simulink library "LocalLib"  (R2015b)
settings: Solver=VariableStepAuto  StartTime=0.0  StopTime=10.0  RelTol=1e-3
values from neighbouring files (symbols this model uses):
  Im = 5e-6    (= 5e-06)    [Params.m]
  Kfr = 5.0e-6    (= 5e-06)    [Params.m]
  KfrOffset = 1.0e-6    (= 1e-06)    [Params.m]
  Ki = (Tq_stall/I_stall)    (= 0.0037456445993)    [MotorModel_Mabuchi_RS_540.m]    (also in Params.m = 0.0041)
  Kv = (Vdc_nom - (I_nl*R_winding))/Om_nl    (= 0.00375385553259)    [MotorModel_Mabuchi_RS_540.m]    (also in Params.m = 0.0039)
  Lm = 1e-5    (= 1e-05)    [Params.m]
  Rm = 0.1672    [Params.m]
libraries: simulink x1
settings Model: Creator=jje  LastModifiedBy=jje

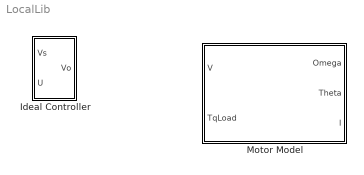
== system LocalLib ==
  Ideal Controller : Subsystem
  Motor Model : Subsystem

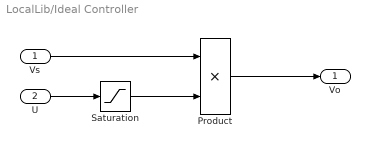
== system LocalLib/Ideal Controller ==
  Vs : Inport
  U : Inport  Port=2
  Product : Product
  Saturation : Saturate  UpperLimit=1  LowerLimit=-1
  Vo : Outport
  wires:
  Vs/1 -> Product/1
  Product/1 -> Vo/1
  U/1 -> Saturation/1
  Saturation/1 -> Product/2

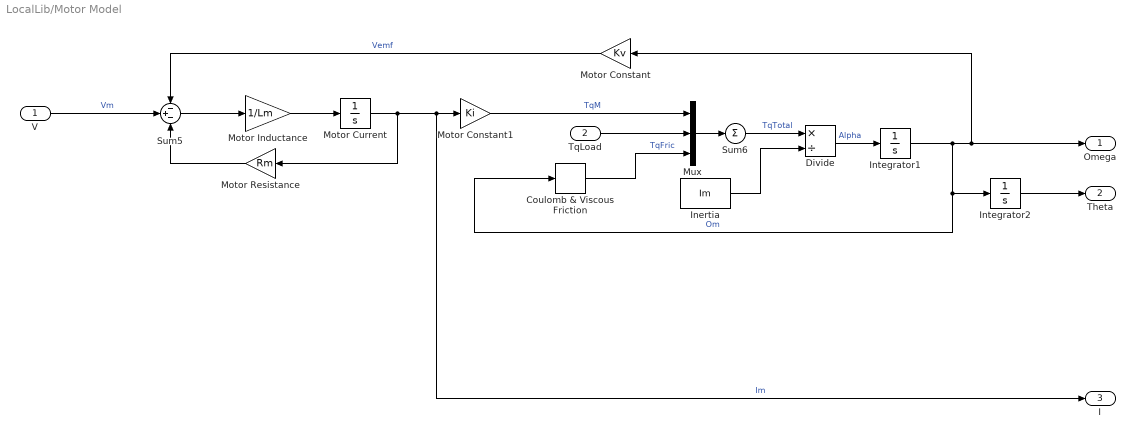
== system LocalLib/Motor Model ==
  V : Inport
  TqLoad : Inport  Port=2
  Coulomb & Viscous Friction : simulink/Discontinuities/Coulomb & Viscous Friction  offset=-KfrOffset  gain=-Kfr
  Divide : Product  Inputs=*/
  Inertia : Constant  Value=Im
  Integrator1 : Integrator
  Integrator2 : Integrator  WrapState=on  WrappedStateUpperValue=2*pi  WrappedStateLowerValue=0
  Motor Constant : Gain  Gain=Kv
  Motor Constant1 : Gain  Gain=Ki
  Motor Current : Integrator
  Motor Inductance : Gain  Gain=1/Lm
  Motor Resistance : Gain  Gain=Rm
  Mux : Mux  Inputs=3
  Sum5 : Sum  Inputs=-+-
  Sum6 : Sum  Inputs=1
  Omega : Outport
  Theta : Outport  Port=2
  I : Outport  Port=3
  wires:
  Motor Constant/1 -> Sum5/1  "Vemf"
  Motor Constant1/1 -> Mux/1  "TqM"
  Motor Resistance/1 -> Sum5/3
  Sum6/1 -> Divide/1  "TqTotal"
  Integrator1/1 -> Coulomb & Viscous Friction/1, Integrator2/1, Omega/1, Motor Constant/1  "Om"
  Divide/1 -> Integrator1/1  "Alpha"
  Inertia/1 -> Divide/2
  Mux/1 -> Sum6/1
  Coulomb & Viscous Friction/1 -> Mux/3  "TqFric"
  V/1 -> Sum5/2  "Vm"
  Motor Inductance/1 -> Motor Current/1
  Sum5/1 -> Motor Inductance/1
  Motor Current/1 -> I/1, Motor Constant1/1, Motor Resistance/1  "Im"
  TqLoad/1 -> Mux/2
  Integrator2/1 -> Theta/1
